simulink model "ECT_harness"  (Simulink 7.7)
settings: Solver=FixedStepDiscrete  SolverMode=SingleTasking  StartTime=0.0  StopTime=100  FixedStep=0.1  RelTol=1e-3
InitFcn:
  | if signalbuilder('ECT_harness/Signal_Builder','activegroup') == 4
  |   CD_SHUTDOWN_FUNCTION.DataType = 'uint8';
  |   CD_SHUTDOWN_FUNCTION.Value = 255;
  | else
  |   CD_SHUTDOWN_FUNCTION.DataType = 'uint8';
  |   CD_SHUTDOWN_FUNCTION.Value = 0;
  | end
  | 
  | if signalbuilder('ECT_harness/Signal_Builder','activegroup') == 7
  |   CD_ECT_FUNCTION.DataType = 'uint8';
  |   CD_ECT_FUNCTION.Value = 255;
  | else
  |   CD_ECT_FUNCTION.DataType = 'uint8';
  |   CD_ECT_FUNCTION.Value = 0;
  | end
  | 
  | if signalbuilder('ECT_harness/Signal_Builder','activegroup') == 8
  |   CD_ECU_FUNCTION.DataType = 'uint8';
  |   CD_ECU_FUNCTION.Value = 0;
  | else
  |   CD_ECU_FUNCTION.DataType = 'uint8';
  |   CD_ECU_FUNCTION.Value = 255;
  | end
undefined symbols (not defined in the file): CD_ECT_FILTER_GAIN, MXGTW_ECTGAUGE, MXGTW_ECTSNDINPUT, MXGTW_ECTSNDOUTPUT, NON_FUNCTIONAL, sigbuilder_block, srate100
libraries: MX_Library x4, simulink x1
CloseFcn:
  | rtwprivate ssgencode ModelCloseRequest sle_main_controller
settings Model: Creator=smindema  LastModifiedBy=aliebel  RecordCoverage=on  CovMetricSettings=dcmtw  CovCumulativeReport=on  CovModelRefEnable=off
settings MATStruct: SampleTime=0.01  Offset=0  Priority=[1.0]
settings DataIOCC: LimitDataPoints=off  SaveOutput=off  SaveTime=off
settings OptimizationCC: BlockReduction=off  InlineParams=on  ExpressionFolding=off  StateBitsets=on  DataBitsets=on  UseTempVars=on  InitFltsAndDblsToZero=on  NoFixptDivByZeroProtection=on  EfficientFloat2IntCast=on  OptimizeModelRefInitCode=on
settings DebuggingCC: SaveWithParameterizedLinksMsg=none  MultiTaskDSMMsg=warning  MultiTaskCondExecSysMsg=none  IntegerOverflowMsg=none  ModelReferenceCSMismatchMessage=warning
settings HardwareCC: ProdBitPerInt=16  ProdBitPerPointer=16  ProdIntDivRoundTo=Floor  ProdEndianess=BigEndian  ProdWordSize=16  ProdHWDeviceType=Motorola HC12
settings ModelReferenceCC: ModelReferenceNumInstancesAllowed=Single
settings RTWCC: SystemTargetFile=ert.tlc  GenCodeOnly=on  TemplateMakefile=ert_default_tmf  Description=Real-Time Workshop Embedded Coder (no auto configuration)  GenerateReport=on  RetainRTWFile=on  ProcessScript=ert_make_rtw_hook  IncludeHyperlinkInReport=on  LaunchReport=on  IncludeERTFirstTime=on
settings RTWCC: CustomHeaderCode=|
  | #include "cpp_req_defines.h"
  | #include "hw_fin.h"
  | #include "cdata.h"
settings CodeAppCC: IgnoreCustomStorageClasses=off  DefineNamingRule=UpperCase
settings ERTTargetCC: TargetFcnLib=ansi_tfl_tmw.mat  FunctionExecutionProfile=off  MultiwordLength=2048  GenerateSampleERTMain=on  IncludeMdlTerminateFcn=off  SupportAbsoluteTime=off  SupportNonFinite=off  SupportComplex=off  PurelyIntegerCode=on  ERTCustomFileTemplate=gen_rtw_req_defines_h.tlc  GlobalDataDefinition=InSeparateSourceFile  GlobalDataReference=InSeparateHeaderFile  ConvertIfToSwitch=off

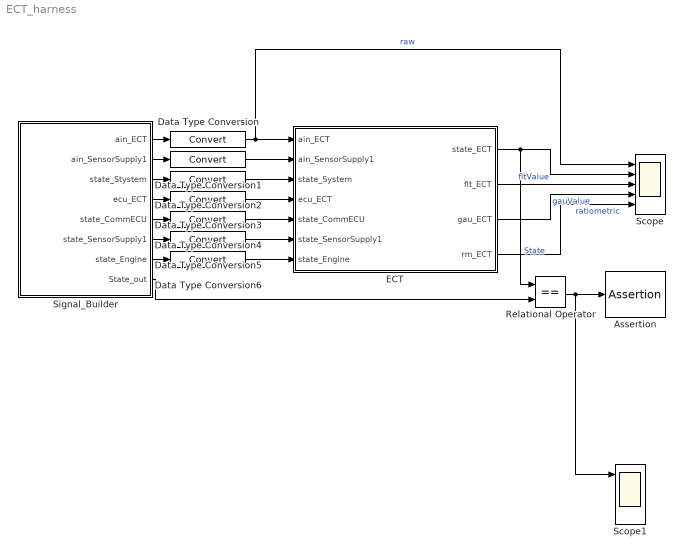
== system ECT_harness ==
  Assertion : Assertion  Enabled=off
  Data Type Conversion : DataTypeConversion  RndMeth=Nearest
  Data Type Conversion{1..6} (6 alike) : DataTypeConversion
  ECT : Subsystem  TreatAsAtomicUnit=on  SystemSampleTime=srate100  RTWFileName=mod_Inputs
      settings: RTWSystemCode=Function  RTWFcnNameOpts=Use subsystem name  RTWFileNameOpts=User specified
  Relational Operator : RelationalOperator  Operator===  OutDataTypeStr=boolean
  Scope : Scope  NumInputPorts=5
      settings: TimeRange=100  YMin=0~7.5~0~0~0  YMax=800~22.5~300~275~900  MaxDataPoints=50000
  Scope1 : Scope  NumInputPorts=5
      settings: TimeRange=100  YMin=0~7.5~0~0~0  YMax=800~22.5~300~275~900  MaxDataPoints=50000
  Signal_Builder : Subsystem  Tag=STV Subsys  LoadFcn=sigbuilder_block('load');  StartFcn=sigbuilder_block('start');  StopFcn=sigbuilder_block('stop');  ClipboardFcn=sigbuilder_block('clipboard');  mask(Sigbuilder block){}
      mask help: Sigbuilder GUI
      mask init:
      | if ~strcmp(get_param(bdroot(gcbh),'SimulationStatus'),'stopped') tuvar = sigbuilder_block('maskInit'); end
      settings: CopyFcn=sigbuilder_block('copy');  DeleteFcn=sigbuilder_block('delete');  ModelCloseFcn=sigbuilder_block('modelClose');  PreSaveFcn=sigbuilder_block('preSave');  NameChangeFcn=sigbuilder_block('namechange');  OpenFcn=sigbuilder_block('open',[1527.75 183 1200 618.75 ]);  CloseFcn=sigbuilder_block('close');
      mask Display: plot(0,0,100,100,[10,10,40,40,10],[80,20,20,80,80],[40,10],[50,50], [40,27,10],[65,72,56],[40,25,25,10],[28,28,43,43]);
  wires:
  ECT/1(state_ECT) -> Scope/2, Relational Operator/1  "State"
  ECT/2(flt_ECT) -> Scope/3  "fltValue"
  ECT/3(gau_ECT) -> Scope/4  "gauValue"
  Signal_Builder/2(ain_SensorSupply1) -> Data Type Conversion1/1
  Data Type Conversion/1 -> Scope/1, ECT/1(ain_ECT)  "raw"
  Data Type Conversion1/1 -> ECT/2(ain_SensorSupply1)
  Data Type Conversion2/1 -> ECT/3(state_System)
  Signal_Builder/1(ain_ECT) -> Data Type Conversion/1
  Data Type Conversion3/1 -> ECT/4(ecu_ECT)
  Data Type Conversion4/1 -> ECT/5(state_CommECU)
  Signal_Builder/8(State_out) -> Relational Operator/2
  Relational Operator/1 -> Assertion/1, Scope1/1
  ECT/4(rm_ECT) -> Scope/5  "ratiometric"
  Signal_Builder/3(state_Stystem) -> Data Type Conversion2/1
  Signal_Builder/4(ecu_ECT) -> Data Type Conversion3/1
  Signal_Builder/5(state_CommECU) -> Data Type Conversion4/1
  Signal_Builder/6(state_SensorSupply1) -> Data Type Conversion5/1
  Signal_Builder/7(state_Engine) -> Data Type Conversion6/1
  Data Type Conversion5/1 -> ECT/6(state_SensorSupply1)
  Data Type Conversion6/1 -> ECT/7(state_Engine)

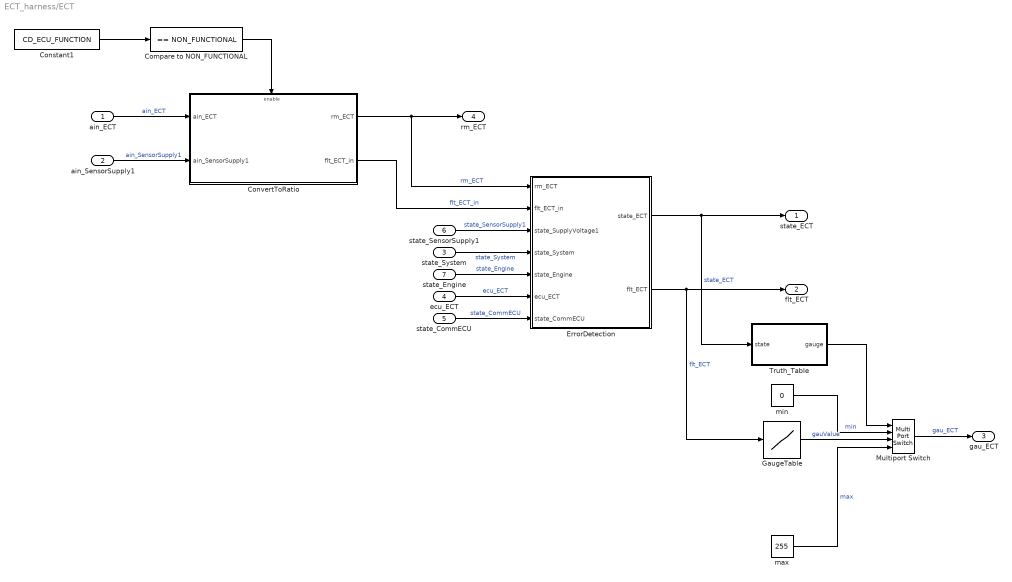
== system ECT_harness/ECT ==
  ain_ECT : Inport  OutDataTypeStr=uint16
  ain_SensorSupply1 : Inport  Port=2  OutDataTypeStr=uint16
  state_System : Inport  Port=3
  ecu_ECT : Inport  Port=4  OutDataTypeStr=uint16
  state_CommECU : Inport  Port=5
  state_SensorSupply1 : Inport  Port=6  OutDataTypeStr=uint8
  state_Engine : Inport  Port=7
  Compare to NON_FUNCTIONAL : simulink/Logic and Bit Operations/Compare To Constant  SystemSampleTime=-1  relop===  const=NON_FUNCTIONAL  LogicOutDataTypeMode=boolean  ZeroCross=off
  Constant1 : Constant  Value=CD_ECU_FUNCTION  OutDataTypeStr=uint8
  ConvertToRatio : Subsystem
  ErrorDetection : Stateflow chart  TreatAsAtomicUnit=on
  GaugeTable : Lookup  InputValues=[0:340]  Table=MXGTW_ECTGAUGE  LookUpMeth=Use Input Nearest  OutDataTypeStr=uint16  RndMeth=Zero  SaturateOnIntegerOverflow=on
      settings: AttributesFormatString=input = %<InputValues>\noutput = %<OutputValues>\nlookup = %<LookUpMeth>\nrounding = %<RndMeth>
  Multiport Switch : MultiPortSwitch  zeroidx=off  OutDataTypeStr=uint16
  Truth_Table : Stateflow chart  TreatAsAtomicUnit=on
  max : Constant  Value=255  OutDataTypeStr=uint16
  min : Constant  Value=0  OutDataTypeStr=uint16
  state_ECT : Outport
  flt_ECT : Outport  Port=2
  gau_ECT : Outport  Port=3
  rm_ECT : Outport  Port=4
  wires:
  ErrorDetection/1(state_ECT) -> state_ECT/1, Truth_Table/1(state)  "state_ECT"
  state_SensorSupply1/1 -> ErrorDetection/3(state_SupplyVoltage1)  "state_SensorSupply1"
  ConvertToRatio/1(rm_ECT) -> rm_ECT/1, ErrorDetection/1(rm_ECT)  "rm_ECT"
  state_System/1 -> ErrorDetection/4(state_System)  "state_System"
  state_Engine/1 -> ErrorDetection/5(state_Engine)  "state_Engine"
  Multiport Switch/1 -> gau_ECT/1  "gau_ECT"
  GaugeTable/1 -> Multiport Switch/3  "gauValue"
  min/1 -> Multiport Switch/2  "min"
  max/1 -> Multiport Switch/4  "max"
  Truth_Table/1(gauge) -> Multiport Switch/1
  ErrorDetection/2(flt_ECT) -> flt_ECT/1, GaugeTable/1  "flt_ECT"
  ain_ECT/1 -> ConvertToRatio/1(ain_ECT)  "ain_ECT"
  ain_SensorSupply1/1 -> ConvertToRatio/2(ain_SensorSupply1)  "ain_SensorSupply1"
  ConvertToRatio/2(flt_ECT_in) -> ErrorDetection/2(flt_ECT_in)  "flt_ECT_in"
  Constant1/1 -> Compare to NON_FUNCTIONAL/1
  ecu_ECT/1 -> ErrorDetection/6(ecu_ECT)  "ecu_ECT"
  state_CommECU/1 -> ErrorDetection/7(state_CommECU)  "state_CommECU"
  Compare to NON_FUNCTIONAL/1 -> ConvertToRatio/Enable

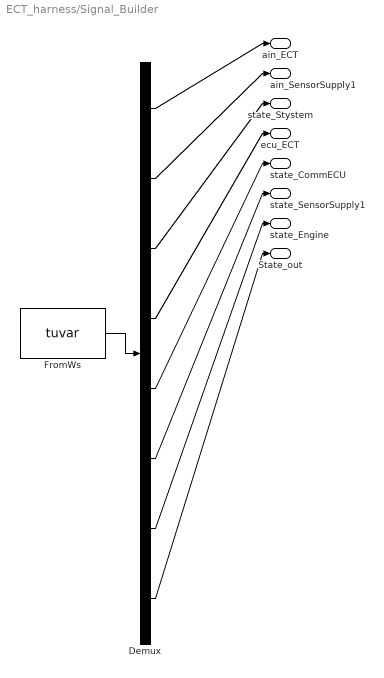
== system ECT_harness/Signal_Builder ==
  Demux : Demux  Tag=STV Demux  Outputs=8
  FromWs : FromWorkspace  Tag=STV FromWs  VariableName=tuvar  SampleTime=0  SigBuilderData=DataTag0  VnvData=DataTag1
      SigBuilderData=|
      | common.afterFinalStr = 'Extrapolate'
      | common.sampleTime = 0
      | dataSet(1).timeRange = [0 100]
      | dataSet(1).name = 'T1-OORL'
      | dataSet(2).timeRange = [0 100]
      | dataSet(2).name = 'T2-OORH'
      | dataSet(3).timeRange = [0 100]
      | dataSet(3).name = 'T3-High'
      | dataSet(4).timeRange = [0 100]
      | dataSet(4).name = 'T4-ExHigh'
      | dataSet(5).timeRange = [0 100]
      | dataSet(5).name = 'T5-Shutdown'
      | dataSet(6).timeRange = [0 100]
      | dataSet(6).name = 'T6-Cold'
      | dataSet(7).timeRange = [0 100]
      | dataSet(7).name = 'T7-NON_FUNC'
      | dataSet(8).timeRange = [0 100]
      | dataSet(8).name = 'T8-ECU'
      | sbobj.Groups(1).Name = 'T1-OORL'
      | sbobj.Groups(1).Signals(1).Name = 'ain_ECT'
      | sbobj.Groups(1).Signals(1).XData = [0 1.4 1.4 2.4 2.4 15.5 15.5 20 20 60.9 60.9 61.5 61.5 71.3 71.3 95.7 95.7 100]
      | sbobj.Groups(1).Signals(1).YData = [30 30 495 495 80 80 505 505 80 80 490 490 80 80 740 740 80 80]
      | sbobj.Groups(1).Signals(2).Name = 'ain_SensorSupply1'
      | sbobj.Groups(1).Signals(2).XData = [0 100]
      | sbobj.Groups(1).Signals(2).YData = [875 875]
      | sbobj.Groups(1).Signals(3).Name = 'state_Stystem'
      | sbobj.Groups(1).Signals(3).XData = [0 0.6 0.6 100]
      | sbobj.Groups(1).Signals(3).YData = [0 0 1 1]
      | sbobj.Groups(1).Signals(4).Name = 'ecu_ECT'
      | sbobj.Groups(1).Signals(4).XData = [0 100]
      | sbobj.Groups(1).Signals(4).YData = [0 0]
      | sbobj.Groups(1).Signals(5).Name = 'state_CommECU'
      | sbobj.Groups(1).Signals(5).XData = [0 100]
      | sbobj.Groups(1).Signals(5).YData = [0 0]
      | sbobj.Groups(1).Signals(6).Name = 'state_SensorSupply1'
      | sbobj.Groups(1).Signals(6).XData = [0 8 8 10.7 10.7 65.4 65.4 66.1 66.1 100]
      | sbobj.Groups(1).Signals(6).YData = [8 8 21 21 8 8 21 21 8 8]
      | sbobj.Groups(1).Signals(7).Name = 'state_Engine'
      | sbobj.Groups(1).Signals(7).XData = [0 71.8 71.8 100]
      | sbobj.Groups(1).Signals(7).YData = [0 0 3 3]
      | sbobj.Groups(1).Signals(8).Name = 'State_out'
      | sbobj.Groups(1).Signals(8).XData = [0 52.9 52.9 83.2 83.2 100]
      | sbobj.Groups(1).Signals(8).YData = [8 8 22 22 11 11]
      | sbobj.Groups(2).Name = 'T2-OORH'
      | sbobj.Groups(2).Signals(1).Name = 'ain_ECT'
      | sbobj.Groups(2).Signals(1).XData = [0 1.4 1.4 2.4 2.4 15.5 15.5 20 20 60.9 60.9 61.5 61.5 68.7 68.7 95.2 95.2 100]
      | sbobj.Groups(2).Signals(1).YData = [895 895 495 495 890 890 505 505 920 920 490 490 920 920 715 715 930 930]
      | sbobj.Groups(2).Signals(2).Name = 'ain_SensorSupply1'
      | sbobj.Groups(2).Signals(2).XData = [0 8.8 8.8 8.9 8.9 100]
      | sbobj.Groups(2).Signals(2).YData = [850 850 10 10 850 850]
      | sbobj.Groups(2).Signals(3).Name = 'state_Stystem'
      | sbobj.Groups(2).Signals(3).XData = [0 100]
      | sbobj.Groups(2).Signals(3).YData = [1 1]
      | sbobj.Groups(2).Signals(4).Name = 'ecu_ECT'
      | sbobj.Groups(2).Signals(4).XData = [0 100]
      | sbobj.Groups(2).Signals(4).YData = [0 0]
      | sbobj.Groups(2).Signals(5).Name = 'state_CommECU'
      | sbobj.Groups(2).Signals(5).XData = [0 100]
      | sbobj.Groups(2).Signals(5).YData = [0 0]
      | sbobj.Groups(2).Signals(6).Name = 'state_SensorSupply1'
      | sbobj.Groups(2).Signals(6).XData = [0 8 8 10.7 10.7 65.4 65.4 66.1 66.1 100]
      | sbobj.Groups(2).Signals(6).YData = [8 8 21 21 8 8 19.8 19.8 8 8]
      | sbobj.Groups(2).Signals(7).Name = 'state_Engine'
      | sbobj.Groups(2).Signals(7).XData = [0 69 69 100]
      | sbobj.Groups(2).Signals(7).YData = [0 0 3 3]
      | sbobj.Groups(2).Signals(8).Name = 'State_out'
      | sbobj.Groups(2).Signals(8).XData = [0 51.1 51.1 80.7 80.7 100]
      | sbobj.Groups(2).Signals(8).YData = [8 8 21 21 11 11]
      | sbobj.Groups(3).Name = 'T3-High'
      | sbobj.Groups(3).Signals(1).Name = 'ain_ECT'
      | sbobj.Groups(3).Signals(1).XData = [0 14 22 22 23.4 23.4 26.2 26.2 70 70 70.1 70.1 84.8 84.8 86 86 100]
      | sbobj.Groups(3).Signals(1).YData = [580 580 695 693 693 560 560 693 693 60 200 693 693 480 480 693 693]
      | sbobj.Groups(3).Signals(2).Name = 'ain_SensorSupply1'
      | sbobj.Groups(3).Signals(2).XData = [0 100]
      | sbobj.Groups(3).Signals(2).YData = [850 850]
      | sbobj.Groups(3).Signals(3).Name = 'state_Stystem'
      | sbobj.Groups(3).Signals(3).XData = [0 100]
      | sbobj.Groups(3).Signals(3).YData = [1 1]
      | sbobj.Groups(3).Signals(4).Name = 'ecu_ECT'
      | sbobj.Groups(3).Signals(4).XData = [0 100]
      | sbobj.Groups(3).Signals(4).YData = [0 0]
      | sbobj.Groups(3).Signals(5).Name = 'state_CommECU'
      | sbobj.Groups(3).Signals(5).XData = [0 100]
      | sbobj.Groups(3).Signals(5).YData = [0 0]
      | sbobj.Groups(3).Signals(6).Name = 'state_SensorSupply1'
      | sbobj.Groups(3).Signals(6).XData = [0 100]
      | sbobj.Groups(3).Signals(6).YData = [8 8]
      | sbobj.Groups(3).Signals(7).Name = 'state_Engine'
      | sbobj.Groups(3).Signals(7).XData = [0 39.9 39.9 48.8 48.8 54.9 54.9 100]
      | sbobj.Groups(3).Signals(7).YData = [3 3 1 1 2 2 3 3]
      | sbobj.Groups(3).Signals(8).Name = 'State_out'
      | sbobj.Groups(3).Signals(8).XData = [0 34.5 34.5 45 45 60 60 100]
      | sbobj.Groups(3).Signals(8).YData = [8 8 10 10 8 8 10 10]
      | sbobj.Groups(4).Name = 'T4-ExHigh'
      | sbobj.Groups(4).Signals(1).Name = 'ain_ECT'
      | sbobj.Groups(4).Signals(1).XData = [0 14 22 23.4 23.4 26.2 26.2 76.6 76.6 77 77 84.8 84.8 86 86 94.6 94.6 100]
      | sbobj.Groups(4).Signals(1).YData = [580 580 720 720 560 560 720 720 60 200 720 720 480 480 693 693 1090 1090]
      | sbobj.Groups(4).Signals(2).Name = 'ain_SensorSupply1'
      | sbobj.Groups(4).Signals(2).XData = [0 100]
      | sbobj.Groups(4).Signals(2).YData = [850 850]
      | sbobj.Groups(4).Signals(3).Name = 'state_Stystem'
      | sbobj.Groups(4).Signals(3).XData = [0 100]
      | sbobj.Groups(4).Signals(3).YData = [1 1]
      | sbobj.Groups(4).Signals(4).Name = 'ecu_ECT'
      | sbobj.Groups(4).Signals(4).XData = [0 100]
      | sbobj.Groups(4).Signals(4).YData = [0 0]
      | sbobj.Groups(4).Signals(5).Name = 'state_CommECU'
      | sbobj.Groups(4).Signals(5).XData = [0 100]
      | sbobj.Groups(4).Signals(5).YData = [0 0]
      | sbobj.Groups(4).Signals(6).Name = 'state_SensorSupply1'
      | sbobj.Groups(4).Signals(6).XData = [0 80.5 80.5 81.9 81.9 100]
      | sbobj.Groups(4).Signals(6).YData = [8 8 21 21 8 8]
      | sbobj.Groups(4).Signals(7).Name = 'state_Engine'
      | sbobj.Groups(4).Signals(7).XData = [0 46.4 46.4 53.9 53.9 100]
      | sbobj.Groups(4).Signals(7).YData = [3 3 1 1 3 3]
      | sbobj.Groups(4).Signals(8).Name = 'State_out'
      | sbobj.Groups(4).Signals(8).XData = [0 37.7 37.7 51.6 51.6 64.1 64.1 80.5 80.5 94.5 94.5 100]
      | sbobj.Groups(4).Signals(8).YData = [8 8 11 11 8 8 11 11 8 8 10 10]
      | sbobj.Groups(5).Name = 'T5-Shutdown'
      | sbobj.Groups(5).Signals(1).Name = 'ain_ECT'
      | sbobj.Groups(5).Signals(1).XData = [0 14 22 33.9 33.9 35.7 35.7 81 81 82.3 82.3 85 85 86.6 86.6 88.3 88.3 88.9 88.9 100]
      | sbobj.Groups(5).Signals(1).YData = [580 580 720 720 570 570 720 720 480 480 720 720 0 0 720 720 920 920 720 720]
      | sbobj.Groups(5).Signals(2).Name = 'ain_SensorSupply1'
      | sbobj.Groups(5).Signals(2).XData = [0 100]
      | sbobj.Groups(5).Signals(2).YData = [850 850]
      | sbobj.Groups(5).Signals(3).Name = 'state_Stystem'
      | sbobj.Groups(5).Signals(3).XData = [0 95.7 95.7 98.1 98.1 100]
      | sbobj.Groups(5).Signals(3).YData = [1 1 3 3 1 1]
      | sbobj.Groups(5).Signals(4).Name = 'ecu_ECT'
      | sbobj.Groups(5).Signals(4).XData = [0 100]
      | sbobj.Groups(5).Signals(4).YData = [0 0]
      | sbobj.Groups(5).Signals(5).Name = 'state_CommECU'
      | sbobj.Groups(5).Signals(5).XData = [0 100]
      | sbobj.Groups(5).Signals(5).YData = [0 0]
      | sbobj.Groups(5).Signals(6).Name = 'state_SensorSupply1'
      | sbobj.Groups(5).Signals(6).XData = [0 100]
      | sbobj.Groups(5).Signals(6).YData = [8 8]
      | sbobj.Groups(5).Signals(7).Name = 'state_Engine'
      | sbobj.Groups(5).Signals(7).XData = [0 40.9 40.9 47.3 47.3 100]
      | sbobj.Groups(5).Signals(7).YData = [3 3 1 1 3 3]
      | sbobj.Groups(5).Signals(8).Name = 'State_out'
      | sbobj.Groups(5).Signals(8).XData = [0 31.6 31.6 46.2 46.2 57.5 57.5 77.7 77.7 95.7 95.7 100]
      | sbobj.Groups(5).Signals(8).YData = [8 8 11 11 8 8 11 11 15 15 8 8]
      | sbobj.Groups(6).Name = 'T6-Cold'
      | sbobj.Groups(6).Signals(1).Name = 'ain_ECT'
      | sbobj.Groups(6).Signals(1).XData = [0 12.1 12.1 14.5 14.5 20.8 20.8 34.6 34.6 35.8 35.8 100]
      | sbobj.Groups(6).Signals(1).YData = [504 504 364.637 364.601 500 500 364.376 363.962 500 500 363.884 362]
      | sbobj.Groups(6).Signals(2).Name = 'ain_SensorSupply1'
      | sbobj.Groups(6).Signals(2).XData = [0 100]
      | sbobj.Groups(6).Signals(2).YData = [850 850]
      | sbobj.Groups(6).Signals(3).Name = 'state_Stystem'
      | sbobj.Groups(6).Signals(3).XData = [0 69.7 69.7 71.9 71.9 100]
      | sbobj.Groups(6).Signals(3).YData = [1 1 3 3 1 1]
      | sbobj.Groups(6).Signals(4).Name = 'ecu_ECT'
      | sbobj.Groups(6).Signals(4).XData = [0 100]
      | sbobj.Groups(6).Signals(4).YData = [0 0]
      | sbobj.Groups(6).Signals(5).Name = 'state_CommECU'
      | sbobj.Groups(6).Signals(5).XData = [0 100]
      | sbobj.Groups(6).Signals(5).YData = [0 0]
      | sbobj.Groups(6).Signals(6).Name = 'state_SensorSupply1'
      | sbobj.Groups(6).Signals(6).XData = [0 65.3 65.3 67.2 67.2 100]
      | sbobj.Groups(6).Signals(6).YData = [8 8 21 21 8 8]
      | sbobj.Groups(6).Signals(7).Name = 'state_Engine'
      | sbobj.Groups(6).Signals(7).XData = [0 39.9 39.9 55.7 55.7 100]
      | sbobj.Groups(6).Signals(7).YData = [3 3 1 1 3 3]
      | sbobj.Groups(6).Signals(8).Name = 'State_out'
      | sbobj.Groups(6).Signals(8).XData = [0 26.1 26.1 45 45 60.8 60.8 65.3 65.3 77.1 77.1 100]
      | sbobj.Groups(6).Signals(8).YData = [8 8 12 12 8 8 12 12 8 8 12 12]
      | sbobj.Groups(7).Name = 'T7-NON_FUNC'
      | sbobj.Groups(7).Signals(1).Name = 'ain_ECT'
      | sbobj.Groups(7).Signals(1).XData = [0 12.1 12.1 14.5 14.5 20.8 20.8 34.6 34.6 35.8 35.8 100]
      | sbobj.Groups(7).Signals(1).YData = [504 504 364.637 364.601 500 500 364.376 363.962 500 500 363.884 362]
      | sbobj.Groups(7).Signals(2).Name = 'ain_SensorSupply1'
      | sbobj.Groups(7).Signals(2).XData = [0 100]
      | sbobj.Groups(7).Signals(2).YData = [850 850]
      | sbobj.Groups(7).Signals(3).Name = 'state_Stystem'
      | sbobj.Groups(7).Signals(3).XData = [0 69.7 69.7 71.9 71.9 100]
      | sbobj.Groups(7).Signals(3).YData = [1 1 3 3 1 1]
      | sbobj.Groups(7).Signals(4).Name = 'ecu_ECT'
      | sbobj.Groups(7).Signals(4).XData = [0 100]
      | sbobj.Groups(7).Signals(4).YData = [0 0]
      | sbobj.Groups(7).Signals(5).Name = 'state_CommECU'
      | sbobj.Groups(7).Signals(5).XData = [0 100]
      | sbobj.Groups(7).Signals(5).YData = [0 0]
      | sbobj.Groups(7).Signals(6).Name = 'state_SensorSupply1'
      | sbobj.Groups(7).Signals(6).XData = [0 65.3 65.3 67.2 67.2 100]
      | sbobj.Groups(7).Signals(6).YData = [8 8 21 21 8 8]
      | sbobj.Groups(7).Signals(7).Name = 'state_Engine'
      | sbobj.Groups(7).Signals(7).XData = [0 39.9 39.9 55.7 55.7 100]
      | sbobj.Groups(7).Signals(7).YData = [3 3 1 1 3 3]
      | sbobj.Groups(7).Signals(8).Name = 'State_out'
      | sbobj.Groups(7).Signals(8).XData = [0 34.5 100]
      | sbobj.Groups(7).Signals(8).YData = [8 8 8]
      | sbobj.Groups(8).Name = 'T8-ECU'
      | sbobj.Groups(8).Signals(1).Name = 'ain_ECT'
      | sbobj.Groups(8).Signals(1).XData = [0 12.1 12.1 14.5 14.5 20.8 20.8 34.6 34.6 35.8 35.8 100]
      | sbobj.Groups(8).Signals(1).YData = [504 504 364.637 364.601 500 500 364.376 363.962 500 500 363.884 362]
      | sbobj.Groups(8).Signals(2).Name = 'ain_SensorSupply1'
      | sbobj.Groups(8).Signals(2).XData = [0 100]
      | sbobj.Groups(8).Signals(2).YData = [850 850]
      | sbobj.Groups(8).Signals(3).Name = 'state_Stystem'
      | sbobj.Groups(8).Signals(3).XData = [0 69.7 69.7 71.9 71.9 100]
      | sbobj.Groups(8).Signals(3).YData = [1 1 3 3 1 1]
      | sbobj.Groups(8).Signals(4).Name = 'ecu_ECT'
      | sbobj.Groups(8).Signals(4).XData = [0 100]
      | sbobj.Groups(8).Signals(4).YData = [0 0]
      | sbobj.Groups(8).Signals(5).Name = 'state_CommECU'
      | sbobj.Groups(8).Signals(5).XData = [0 42 42 54.9 54.9 100]
      | sbobj.Groups(8).Signals(5).YData = [0 0 4 4 8 8]
      | sbobj.Groups(8).Signals(6).Name = 'state_SensorSupply1'
      | sbobj.Groups(8).Signals(6).XData = [0 65.3 65.3 67.2 67.2 100]
      | sbobj.Groups(8).Signals(6).YData = [8 8 21 21 8 8]
      | sbobj.Groups(8).Signals(7).Name = 'state_Engine'
      | sbobj.Groups(8).Signals(7).XData = [0 39.9 39.9 55.7 55.7 100]
      | sbobj.Groups(8).Signals(7).YData = [3 3 1 1 3 3]
      | sbobj.Groups(8).Signals(8).Name = 'State_out'
      | sbobj.Groups(8).Signals(8).XData = [0 34.5 100]
      | sbobj.Groups(8).Signals(8).YData = [8 8 8]
  ain_ECT : Outport  Tag=STV Outport
  ain_SensorSupply1 : Outport  Tag=STV Outport  Port=2
  state_Stystem : Outport  Tag=STV Outport  Port=3
  ecu_ECT : Outport  Tag=STV Outport  Port=4
  state_CommECU : Outport  Tag=STV Outport  Port=5
  state_SensorSupply1 : Outport  Tag=STV Outport  Port=6
  state_Engine : Outport  Tag=STV Outport  Port=7
  State_out : Outport  Tag=STV Outport  Port=8
  wires:
  FromWs/1 -> Demux/1
  Demux/1 -> ain_ECT/1
  Demux/2 -> ain_SensorSupply1/1
  Demux/3 -> state_Stystem/1
  Demux/4 -> ecu_ECT/1
  Demux/5 -> state_CommECU/1
  Demux/6 -> state_SensorSupply1/1
  Demux/7 -> state_Engine/1
  Demux/8 -> State_out/1

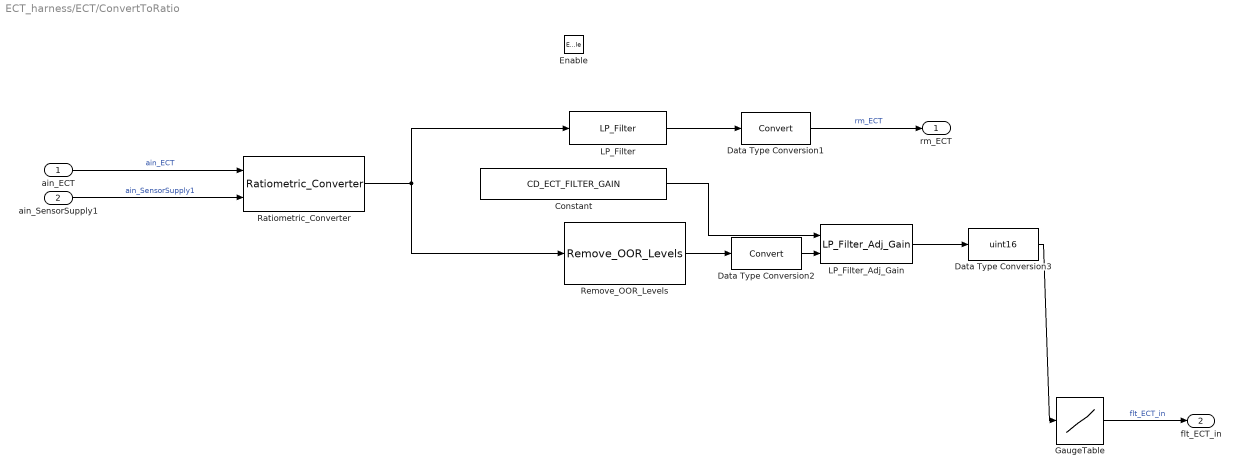
== system ECT_harness/ECT/ConvertToRatio ==
  ain_ECT : Inport  OutDataTypeStr=uint16
  ain_SensorSupply1 : Inport  Port=2  OutDataTypeStr=uint16
  Enable : EnablePort  StatesWhenEnabling=reset  PropagateVarSize=During execution
  Constant : Constant  Value=CD_ECT_FILTER_GAIN  OutDataTypeStr=uint8
  Data Type Conversion1 : DataTypeConversion
  Data Type Conversion2 : DataTypeConversion
  Data Type Conversion3 : DataTypeConversion  OutDataTypeStr=uint16
  GaugeTable : Lookup  InputValues=MXGTW_ECTSNDINPUT  Table=MXGTW_ECTSNDOUTPUT  LookUpMeth=Use Input Nearest  OutDataTypeStr=uint16  RndMeth=Zero  SaturateOnIntegerOverflow=on
      settings: AttributesFormatString=input = %<InputValues>\noutput = %<OutputValues>\nlookup = %<LookUpMeth>\nrounding = %<RndMeth>
  LP_Filter : MX_Library/LP_Filter  SystemSampleTime=-1  GAIN=3
  LP_Filter_Adj_Gain : MX_Library/LP_Filter_Adj_Gain  SystemSampleTime=-1
  Ratiometric_Converter : MX_Library/Ratiometric_Converter  SystemSampleTime=-1  multiplier=1000
  Remove_OOR_Levels : MX_Library/Remove_OOR_Levels  SystemSampleTime=-1  OORL_LEVEL=CD_ECT_OORL  OORH_LEVEL=CD_ECT_OORH
  rm_ECT : Outport  InitialOutput=[0]
  flt_ECT_in : Outport  Port=2  InitialOutput=[0]
  wires:
  ain_ECT/1 -> Ratiometric_Converter/1  "ain_ECT"
  ain_SensorSupply1/1 -> Ratiometric_Converter/2  "ain_SensorSupply1"
  Ratiometric_Converter/1 -> Remove_OOR_Levels/1, LP_Filter/1
  GaugeTable/1 -> flt_ECT_in/1  "flt_ECT_in"
  Data Type Conversion1/1 -> rm_ECT/1  "rm_ECT"
  Remove_OOR_Levels/1 -> Data Type Conversion2/1
  LP_Filter/1 -> Data Type Conversion1/1
  Constant/1 -> LP_Filter_Adj_Gain/1
  Data Type Conversion2/1 -> LP_Filter_Adj_Gain/2
  LP_Filter_Adj_Gain/1 -> Data Type Conversion3/1
  Data Type Conversion3/1 -> GaugeTable/1

== matlab function ECT/Truth_Table ==
  data: state input uint8; gauge output uint8
function gauge = fcn(state)

aVarTruthTableCondition_1 = false;
aVarTruthTableCondition_2 = false;


% OORH

aVarTruthTableCondition_1 = logical(state == 21);

% OORL

aVarTruthTableCondition_2 = logical(state == 22);

if (aVarTruthTableCondition_1)
    aFcnTruthTableAction_3();
elseif (aVarTruthTableCondition_2)
    aFcnTruthTableAction_1();
else % Default
    aFcnTruthTableAction_2();
end

function aFcnTruthTableAction_1()

% Gauge min

gauge = uint8(1);

function aFcnTruthTableAction_2()

% Gauge current

gauge = uint8(2);

function aFcnTruthTableAction_3()

% Gauge max

gauge = uint8(3);

== stateflow chart ECT/ErrorDetection ==
  state SENSOR
    state STATE [parallel]
      settings: executionOrder=2
      state NON_FUNCTIONAL
        en:state_ECT = NORMAL;
      state NORMAL
        state SHUTDOWN
          state SHUTDOWN
            en:state_ECT = SHUTDOWN;
          state DEBOUNCE
            en:debounceCount = 0;
            du:debounceCount++;
          (default) -> SENSOR.STATE.NORMAL.SHUTDOWN.DEBOUNCE
          SENSOR.STATE.NORMAL.SHUTDOWN.DEBOUNCE -> SENSOR.STATE.NORMAL.SHUTDOWN.SHUTDOWN : [(debounceCount >= CD_ECT_DEBOUNCE_SHUTDOWN)]
        state EXTREMELY_HIGH
          state DEBOUNCE
            en:debounceCount = 0;
            du:debounceCount++;
          state EXTREMELY_HIGH
            en:state_ECT = EXTREMELY_HIGH;
          (default) -> SENSOR.STATE.NORMAL.EXTREMELY_HIGH.DEBOUNCE
          SENSOR.STATE.NORMAL.EXTREMELY_HIGH.DEBOUNCE -> SENSOR.STATE.NORMAL.EXTREMELY_HIGH.EXTREMELY_HIGH : [(debounceCount >= CD_ECT_DEBOUNCE_EXTREMELY_HIGH)...
              | || (state_ECT == EXTREMELY_HIGH)]
        state HIGH
          state HIGH
            en:state_ECT = HIGH;
          state DEBOUNCE
            en:debounceCount = 0;
            du:debounceCount++;
          (default) -> SENSOR.STATE.NORMAL.HIGH.DEBOUNCE
          SENSOR.STATE.NORMAL.HIGH.DEBOUNCE -> SENSOR.STATE.NORMAL.HIGH.HIGH : [(debounceCount >= CD_ECT_DEBOUNCE_HIGH)...
              | || (state_ECT == HIGH)]
        state NORMAL
          state DEBOUNCE_NORMAL
            en:debounceCount = 0;
            du:debounceCount++;
          state NORMAL
            en:state_ECT = NORMAL;
          (default) -> SENSOR.STATE.NORMAL.NORMAL.DEBOUNCE_NORMAL
          SENSOR.STATE.NORMAL.NORMAL.DEBOUNCE_NORMAL -> SENSOR.STATE.NORMAL.NORMAL.NORMAL : [(debounceCount >= CD_ECT_DEBOUNCE_NORMAL)...
              | || (state_ECT == NORMAL)]
        state COLD
          state COLD
            en:state_ECT = COLD;
          state DEBOUNCE
            en:debounceCount = 0;
            du:debounceCount++;
          (default) -> SENSOR.STATE.NORMAL.COLD.DEBOUNCE
          SENSOR.STATE.NORMAL.COLD.DEBOUNCE -> SENSOR.STATE.NORMAL.COLD.COLD : [(debounceCount >= CD_ECT_DEBOUNCE_COLD)...
              | || (state_ECT == COLD)]
        SENSOR.STATE.NORMAL.EXTREMELY_HIGH -> SENSOR.STATE.NORMAL.SHUTDOWN [order 2] : [(CD_SHUTDOWN_FUNCTION != NON_FUNCTIONAL)...
            | && (state_ECT == EXTREMELY_HIGH)]
        SENSOR.STATE.NORMAL.SHUTDOWN -> SENSOR.STATE.NORMAL.EXTREMELY_HIGH : [(state_ECT != SHUTDOWN)...
            | && ((flt_ECT_in < (CD_ECT_EXTREMELY_HIGH - CD_TEMPERATURE_HYSTERESIS)) || (state_Engine != ENGINE_RUNNING))]
        SENSOR.STATE.NORMAL.HIGH -> SENSOR.STATE.NORMAL.EXTREMELY_HIGH [order 2] : [(flt_ECT_in >= CD_ECT_EXTREMELY_HIGH)]
        SENSOR.STATE.NORMAL.EXTREMELY_HIGH -> SENSOR.STATE.NORMAL.HIGH [order 1] : [(flt_ECT_in < (CD_ECT_EXTREMELY_HIGH - CD_TEMPERATURE_HYSTERESIS))...
            | || (state_Engine != ENGINE_RUNNING)]
        SENSOR.STATE.NORMAL.HIGH -> SENSOR.STATE.NORMAL.NORMAL [order 1] : [(flt_ECT_in < (CD_ECT_HIGH - CD_TEMPERATURE_HYSTERESIS))...
            | || (state_Engine != ENGINE_RUNNING)]
        SENSOR.STATE.NORMAL.NORMAL -> SENSOR.STATE.NORMAL.HIGH [order 2] : [(flt_ECT_in >= CD_ECT_HIGH)...
            | && (state_Engine == ENGINE_RUNNING)]
        (default) -> SENSOR.STATE.NORMAL.NORMAL
        SENSOR.STATE.NORMAL.NORMAL -> SENSOR.STATE.NORMAL.COLD [order 1] : [(flt_ECT_in <= CD_ECT_COLD)...
            | && (state_Engine == ENGINE_RUNNING)]
        SENSOR.STATE.NORMAL.COLD -> SENSOR.STATE.NORMAL.NORMAL : [(flt_ECT_in > (CD_ECT_COLD + CD_TEMPERATURE_HYSTERESIS))...
            | || (state_Engine != ENGINE_RUNNING)]
      state OUT_OF_RANGE_HIGH
        state DEBOUNCE
          en:debounceCount = 0;
          du:debounceCount++;
        state OORH
          en:state_ECT = OORH;
        (default) -> SENSOR.STATE.OUT_OF_RANGE_HIGH.DEBOUNCE
        SENSOR.STATE.OUT_OF_RANGE_HIGH.DEBOUNCE -> OORH : [(debounceCount >= CD_ECT_DEBOUNCE_OORH)...
            | || (state_ECT == OORH)]
      state OUT_OF_RANGE_LOW
        state DEBOUNCE
          en:debounceCount = 0;
          du:debounceCount++;
        state OORL
          en:state_ECT = OORL;
        (default) -> SENSOR.STATE.OUT_OF_RANGE_LOW.DEBOUNCE
        SENSOR.STATE.OUT_OF_RANGE_LOW.DEBOUNCE -> OORL : [(debounceCount >= CD_ECT_DEBOUNCE_OORL)...
            | || (state_ECT == OORL)]
      (default) -> NON_FUNCTIONAL
      SENSOR.STATE.NORMAL -> NON_FUNCTIONAL [order 1] : [(state_SupplyVoltage1 != NORMAL)...
          | || (state_System != SYS_NORMAL)]
      NON_FUNCTIONAL -> SENSOR.STATE.NORMAL : [(CD_ECT_FUNCTION != NON_FUNCTIONAL)...
          | && (state_SupplyVoltage1 == NORMAL)...
          | && (state_System == SYS_NORMAL)]
      SENSOR.STATE.NORMAL -> OUT_OF_RANGE_HIGH [order 3] : [(rm_ECT >= CD_ECT_OORH)...
          | && (state_ECT != SHUTDOWN)]
      OUT_OF_RANGE_HIGH -> SENSOR.STATE.NORMAL [order 1] : [(rm_ECT < CD_ECT_OORH)]
      SENSOR.STATE.NORMAL -> OUT_OF_RANGE_LOW [order 2] : [(rm_ECT <= CD_ECT_OORL)...
          | && (state_ECT != SHUTDOWN)]
      OUT_OF_RANGE_LOW -> SENSOR.STATE.NORMAL [order 1] : [(rm_ECT > CD_ECT_OORL)]
      OUT_OF_RANGE_HIGH -> NON_FUNCTIONAL [order 2] : [(state_SupplyVoltage1 != NORMAL)...
          | && (state_ECT != OORH)]
      OUT_OF_RANGE_LOW -> NON_FUNCTIONAL [order 2] : [(state_SupplyVoltage1 != NORMAL)...
          | && (state_ECT != OORL)]
    state VALUE [parallel]
      settings: executionOrder=1
      state INIT
        en:flt_ECT = 0;
        (default) -> (junction 56)
        (junction 56) -> (junction 57) [order 1] : [(rm_ECT <= CD_ECT_OORL)...
            | || (rm_ECT >= CD_ECT_OORH)]
        (junction 56) -> (junction 58) [order 2] : {
            | flt_ECT = flt_ECT_in;
            | }
        (junction 57) -> (junction 59) : {
            | flt_ECT = 0;
            | }
        (junction 59) -> (junction 58)
      state NORMAL
        du:flt_ECT = flt_ECT_in;
      (default) -> INIT
      INIT -> SENSOR.VALUE.NORMAL : [(state_System == SYS_NORMAL)]
  state ECU
    state NORMAL
      du:flt_ECT = ecu_ECT;
      state SHUTDOWN
        state SHUTDOWN
          en:state_ECT = SHUTDOWN;
        state DEBOUNCE
          en:debounceCount = 0;
          du:debounceCount++;
        (default) -> ECU.NORMAL.SHUTDOWN.DEBOUNCE
        ECU.NORMAL.SHUTDOWN.DEBOUNCE -> ECU.NORMAL.SHUTDOWN.SHUTDOWN : [(debounceCount >= CD_ECT_DEBOUNCE_SHUTDOWN)]
      state EXTREMELY_HIGH
        state DEBOUNCE
          en:debounceCount = 0;
          du:debounceCount++;
        state EXTREMELY_HIGH
          en:state_ECT = EXTREMELY_HIGH;
        (default) -> ECU.NORMAL.EXTREMELY_HIGH.DEBOUNCE
        ECU.NORMAL.EXTREMELY_HIGH.DEBOUNCE -> ECU.NORMAL.EXTREMELY_HIGH.EXTREMELY_HIGH : [(debounceCount >= CD_ECT_DEBOUNCE_EXTREMELY_HIGH)...
            | || (state_ECT == EXTREMELY_HIGH)]
      state HIGH
        state HIGH
          en:state_ECT = HIGH;
        state DEBOUNCE
          en:debounceCount = 0;
          du:debounceCount++;
        (default) -> ECU.NORMAL.HIGH.DEBOUNCE
        ECU.NORMAL.HIGH.DEBOUNCE -> ECU.NORMAL.HIGH.HIGH : [(debounceCount >= CD_ECT_DEBOUNCE_HIGH)...
            | || (state_ECT == HIGH)]
      state NORMAL
        state DEBOUNCE_NORMAL
          en:debounceCount = 0;
          du:debounceCount++;
        state NORMAL
          en:state_ECT = NORMAL;
        (default) -> ECU.NORMAL.NORMAL.DEBOUNCE_NORMAL
        ECU.NORMAL.NORMAL.DEBOUNCE_NORMAL -> ECU.NORMAL.NORMAL.NORMAL : [(debounceCount >= CD_ECT_DEBOUNCE_NORMAL)...
            | || (state_ECT == NORMAL)]
      state COLD
        state COLD
          en:state_ECT = COLD;
        state DEBOUNCE
          en:debounceCount = 0;
          du:debounceCount++;
        (default) -> ECU.NORMAL.COLD.DEBOUNCE
        ECU.NORMAL.COLD.DEBOUNCE -> ECU.NORMAL.COLD.COLD : [(debounceCount >= CD_ECT_DEBOUNCE_COLD)...
            | || (state_ECT == COLD)]
      ECU.NORMAL.EXTREMELY_HIGH -> ECU.NORMAL.SHUTDOWN [order 2] : [(CD_SHUTDOWN_FUNCTION != NON_FUNCTIONAL)...
          | && (state_ECT == EXTREMELY_HIGH)]
      ECU.NORMAL.SHUTDOWN -> ECU.NORMAL.EXTREMELY_HIGH : [(state_ECT != SHUTDOWN)...
          | && ((flt_ECT < (CD_ECT_EXTREMELY_HIGH - CD_TEMPERATURE_HYSTERESIS)) || (state_Engine != ENGINE_RUNNING))]
      ECU.NORMAL.HIGH -> ECU.NORMAL.EXTREMELY_HIGH [order 2] : [(flt_ECT >= CD_ECT_EXTREMELY_HIGH)]
      ECU.NORMAL.EXTREMELY_HIGH -> ECU.NORMAL.HIGH [order 1] : [(flt_ECT < (CD_ECT_EXTREMELY_HIGH - CD_TEMPERATURE_HYSTERESIS))...
          | || (state_Engine != ENGINE_RUNNING)]
      ECU.NORMAL.NORMAL -> ECU.NORMAL.HIGH [order 2] : [(flt_ECT >= CD_ECT_HIGH)...
          | && (state_Engine == ENGINE_RUNNING)]
      ECU.NORMAL.HIGH -> ECU.NORMAL.NORMAL [order 1] : [(flt_ECT < (CD_ECT_HIGH - CD_TEMPERATURE_HYSTERESIS))...
          | || (state_Engine != ENGINE_RUNNING)]
      (default) -> ECU.NORMAL.NORMAL
      ECU.NORMAL.NORMAL -> ECU.NORMAL.COLD [order 1] : [(flt_ECT <= CD_ECT_COLD)...
          | && (state_Engine == ENGINE_RUNNING)]
      ECU.NORMAL.COLD -> ECU.NORMAL.NORMAL : [(flt_ECT > (CD_ECT_COLD + CD_TEMPERATURE_HYSTERESIS))...
          | || (state_Engine != ENGINE_RUNNING)]
    state NO_COMMUNICATION
      en:flt_ECT = 0;
    (default) -> ECU.NORMAL
    ECU.NORMAL -> NO_COMMUNICATION : [(state_CommECU == NO_COMMUNICATION)]
    NO_COMMUNICATION -> ECU.NORMAL : [(state_CommECU != NO_COMMUNICATION)]
  SENSOR -> ECU : [(CD_ECU_FUNCTION != NON_FUNCTIONAL)]
  (default) -> SENSOR
  data: rm_ECT input uint16; flt_ECT_in input uint16; state_ECT output uint8; state_SupplyVoltage1 input double; CD_ECT_FUNCTION parameter uint8; CD_ECT_OORH parameter uint16; CD_ECT_OORL parameter uint16; CD_ECT_DEBOUNCE_OORH parameter uint16; CD_ECT_DEBOUNCE_OORL parameter uint16; CD_ECT_DEBOUNCE_NORMAL parameter uint16; CD_ECT_DEBOUNCE_HIGH parameter uint16; CD_ECT_DEBOUNCE_COLD parameter uint16; CD_ECT_DEBOUNCE_EXTREMELY_HIGH parameter uint16; CD_ECT_DEBOUNCE_SHUTDOWN parameter uint16; CD_ECT_HIGH parameter uint16; CD_ECT_EXTREMELY_HIGH parameter uint16; CD_ECT_COLD parameter uint16; debounceCount local uint16 =0; CD_SHUTDOWN_FUNCTION parameter uint8; CD_TEMPERATURE_HYSTERESIS parameter uint16; COLD parameter uint8 =12; EXTREMELY_HIGH parameter uint8 =11; HIGH parameter uint8 =10; NON_FUNCTIONAL parameter uint8 =255; NORMAL parameter uint8 =8; OORH parameter uint8 =21; OORL parameter uint8 =22; SHUTDOWN parameter uint8 =15; state_System input uint8; SYS_NORMAL parameter uint8; state_Engine input uint8; ENGINE_RUNNING parameter uint8; flt_ECT output uint16; ecu_ECT input uint16; state_CommECU input uint8; CD_ECU_FUNCTION parameter uint8; NO_COMMUNICATION parameter uint8
